simulink subsystem "GPS_MAX_M10S"  (R2025b)
settings: Solver=VariableStepAuto  StartTime=0.0  StopTime=10.0  RelTol=1e-3
settings Model: Creator=Admin  LastModifiedBy=slee7

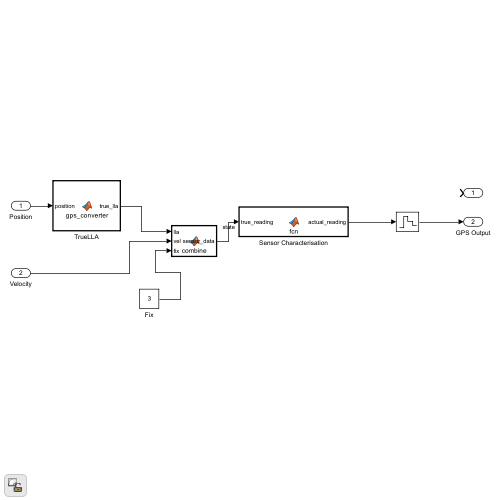
[thumbnail: Simulink's stored preview of the top-level diagram]
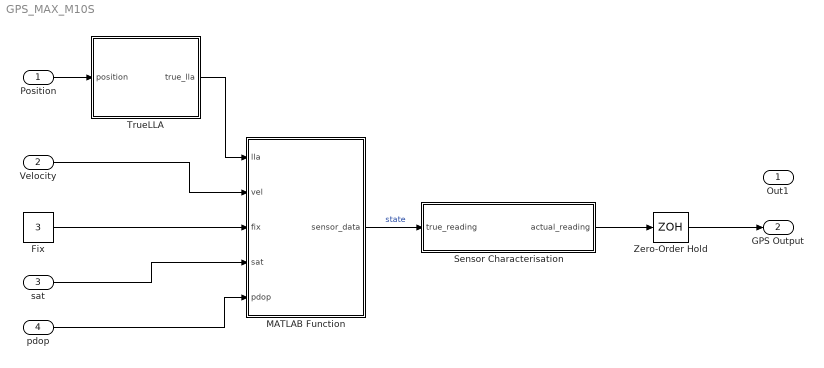
== system GPS_MAX_M10S ==
  Position : Inport
  Velocity : Inport  Port=2
  sat : Inport  Port=3
  pdop : Inport  Port=4
  Fix : Constant  Value=3
  MATLAB Function : MATLAB Function  TreatAsAtomicUnit=on
  Sensor Characterisation : MATLAB Function  TreatAsAtomicUnit=on
  TrueLLA : MATLAB Function  TreatAsAtomicUnit=on
  Zero-Order Hold : ZeroOrderHold  SampleTime=0.1
  Out1 : Outport
  GPS Output : Outport  Port=2
  wires:
  MATLAB Function/1(sensor_data) -> Sensor Characterisation/1(true_reading)  "state"
  Position/1 -> TrueLLA/1(position)
  Zero-Order Hold/1 -> GPS Output/1
  Sensor Characterisation/1(actual_reading) -> Zero-Order Hold/1
  TrueLLA/1(true_lla) -> MATLAB Function/1(lla)
  Velocity/1 -> MATLAB Function/2(vel)
  Fix/1 -> MATLAB Function/3(fix)
  sat/1 -> MATLAB Function/4(sat)
  pdop/1 -> MATLAB Function/5(pdop)

== matlab function GPS_MAX_M10S/MATLAB Function ==
  data: lla input; sensor_data output; vel input; fix input; sat input; pdop input
function sensor_data = combine(lla, vel, fix, sat, pdop)

sensor_data = [lla; vel; fix; sat; pdop];

== matlab function GPS_MAX_M10S/Sensor Characterisation ==
  data: true_reading input; actual_reading output
function actual_reading = fcn(true_reading)
    persistent b_previous
lla, vel, fix, sat, pdop)

    % true reading = [lat; lng; alt; v_n; v_e; v_d; sat; pdop]

    dt = 0.02; % CAN Bus limit 20 ms

    % Bias: Composite Bias = Const + Gauss-Markov Drift
    
        b_const = [0; 0; 0; 0; 0; 0; 0; 0; 0]; % Constant bias
    
        % Drift bias (b = exp^-dt/tau * b_previous + omega)
        
        if isempty(b_previous)
            b_previous = [0 0 0]; 
        end
    
        tau = [83.024; 83.064; 107.711; 0.23726; 0.525419; 0.15266; inf; inf]; % time constant of drift
        q = [3.6570824.861]; % variance on drift
    
        omega = sqrt(q) .* randn(3,1); % omega ~ N(0,q)
        
        b_drift = exp(-dt ./ tau) .* b_previous + omega;
    
        composite_bias = b_const + b_drift; 

    % Noise: Gaussian  

        noise_variance = [1.645664; 1.487596; 1.836378]; 
    
        noise = noise_variance .* randn(3,1); 
    
    % Quantisation:

        quant_step = 0.5; % Quant Step: data sheet
   

    % Reading Processing:

        actual_reading_continuous  = true_reading(:) + composite_bias + noise;

        actual_reading_quantised = quant_step * round(actual_reading_continuous/quant_step);

        actual_reading = actual_reading_quantised; 

end

% Currently Ignoring: 
% Scale_factor_error 
% Misalignment_error

== matlab function GPS_MAX_M10S/TrueLLA ==
  data: position input; true_lla output
function true_lla = gps_converter(position)
% position = [N; E; D] in meters (NED frame, D positive down)
% true_lla  = [lat_deg, lon_deg, h_m]

north = position(1);
east  = position(2);
down  = position(3);

% Fixed reference LLA (degrees, degrees, meters)
lat0 = 51.507351;
lon0 = -0.127758;
h0   = 25;

% WGS84 Earth model
spheroid = wgs84Ellipsoid("meter");

[lat, lon, h] = ned2geodetic(north, east, down, lat0, lon0, h0, spheroid);

true_lla = [lat; lon; h];
end
